simulink model "controller"  (R2021a)
settings: Solver=FixedStepDiscrete  StartTime=0.0  StopTime=10.0  FixedStep=1  RelTol=1e-3  EnableMultiTasking=on
settings Model: DataDictionary=worldDD.sldd  SILPILModeSetting=veronly  ExtModeTrigDuration=2  Creator=Koorosh  LastModifiedBy=Koorosh
settings OptimizationCC: EnhancedBackFolding=on  PassReuseOutputArgsAs=Individual arguments  ZeroExternalMemoryAtStartup=off  ZeroInternalMemoryAtStartup=off  MaxStackSize=64  OptimizeBlockOrder=speed  DifferentSizesBufferReuse=on  OptimizationCustomize=off  EfficientTunableParamExpr=on
settings DebuggingCC: ParameterTunabilityLossMsg=error
settings HardwareCC: ProdBitPerInt=16  ProdBitPerPointer=16  ProdBitPerSizeT=16  ProdBitPerPtrDiffT=16  ProdLargestAtomicFloat=None  ProdWordSize=8  ProdHWDeviceType=Atmel->AVR
settings SFSimCC: MATLABDynamicMemAlloc=off
settings RTWCC: SystemTargetFile=ert.tlc  HardwareBoard=Arduino Uno  GenCodeOnly=on  TemplateMakefile=ert_default_tmf  GenerateReport=on  Toolchain=Arduino AVR  BuildConfiguration=Faster Runs  LaunchReport=on  GenerateWebview=on
settings CodeAppCC: ForceParamTrailComments=on  IgnoreCustomStorageClasses=off  OperatorAnnotations=on  SimulinkDataObjDesc=on  SFDataObjDesc=on  InsertBlockDesc=on
settings ERTTargetCC: SupportContinuousTime=on  SupportVariableSizeSignals=on  ExtModeStaticAllocSize=250

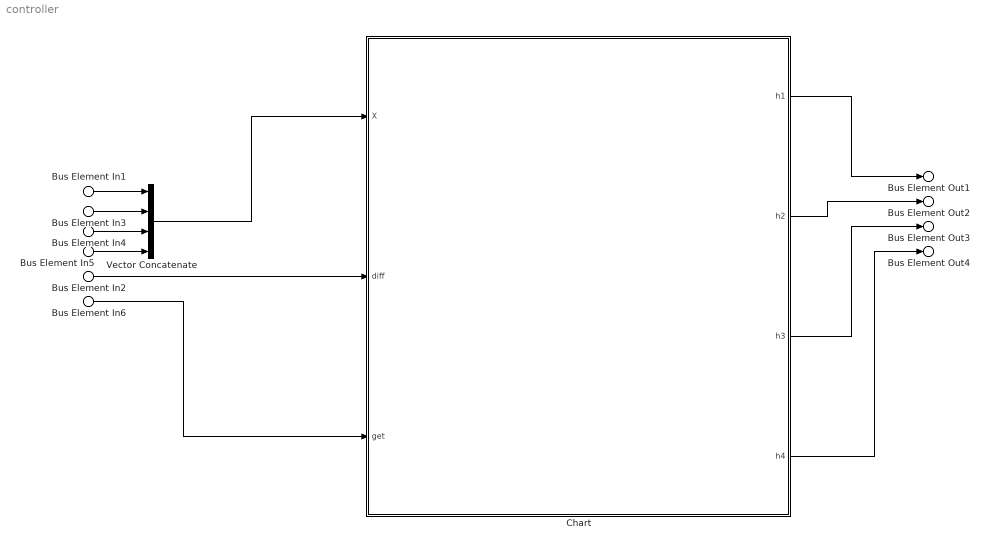
== system controller ==
  Bus Element In1 : Inport  PortName=X  Element=x1
  Bus Element In3 : Inport  PortName=X  Element=x2
  Bus Element In4 : Inport  PortName=X  Element=x3
  Bus Element In5 : Inport  PortName=X  Element=x4
  Bus Element In6 : Inport  Port=2  PortName=C  Element=get
  Bus Element In2 : Inport  Port=2  PortName=C  Element=diff
  Chart : Stateflow chart  TreatAsAtomicUnit=on
  Vector Concatenate : Concatenate  NumInputs=4
  Bus Element Out1 : Outport  PortName=H  Element=h1
  Bus Element Out2 : Outport  PortName=H  Element=h2
  Bus Element Out3 : Outport  PortName=H  Element=h3
  Bus Element Out4 : Outport  PortName=H  Element=h4
  wires:
  Chart/1(h1) -> Bus Element Out1/1
  Chart/2(h2) -> Bus Element Out2/1
  Chart/3(h3) -> Bus Element Out3/1
  Chart/4(h4) -> Bus Element Out4/1
  Bus Element In2/1 -> Chart/2(diff)
  Bus Element In6/1 -> Chart/3(get)
  Bus Element In1/1 -> Vector Concatenate/1
  Bus Element In3/1 -> Vector Concatenate/2
  Bus Element In4/1 -> Vector Concatenate/3
  Bus Element In5/1 -> Vector Concatenate/4
  Vector Concatenate/1 -> Chart/1(X)

== stateflow chart controller/Chart ==
  settings: stateMachineType=MOORE_MACHINE
  state h1h2
    U(1,2);
  state h1h3
    U(1,3);
  state init_state
  state h1h4
    U(1,4);
  state h3h4
    U(3,4);
  state h2h3
    U(2,3);
  state h2h4
    U(2,4);
  h1h2 -> h3h4 [order 2] : [(T(1,3)&T(2,4))|(T(1,4)&T(2,3))]
  h1h3 -> h1h2 [order 1] : [T(3,2)|(T(1,2)&T(3,1))]
  h1h3 -> h1h4 [order 2] : [T(3,4)|(T(1,4)&T(3,1))]
  h1h2 -> h1h3 [order 1] : [T(2,3)|(T(2,1)&T(1,3))]
  h1h4 -> h1h2 [order 4] : [T(4,2)|(T(1,2)&T(4,1))]
  h3h4 -> h1h2 [order 2] : [(T(3,1)&T(4,2))|(T(4,1)&T(3,2))]
  h1h4 -> h1h3 [order 1] : [T(4,3)|(T(4,1)&T(1,3))]
  h3h4 -> h1h3 [order 4] : [T(4,1)|(T(4,3)&T(3,1))]
  h1h2 -> h1h4 [order 5] : [T(2,4)|(T(2,1)&T(1,4))]
  h1h3 -> h3h4 [order 5] : [T(1,4)|(T(3,4)&T(1,3))]
  h2h3 -> h1h2 [order 4] : [T(3,1)|(T(2,1)&T(3,2))]
  h1h2 -> h2h3 [order 4] : [T(1,3)|(T(1,2)&T(2,3))]
  init_state -> h1h2 [order 1] : [h1==1 & h2==1]
  h2h4 -> h1h2 [order 3] : [T(4,1)|(T(2,1)&T(4,2))]
  h1h2 -> h2h4 [order 3] : [T(1,4)|(T(1,2)&T(2,4))]
  h2h3 -> h1h3 [order 3] : [T(2,1)|(T(3,1)&T(2,3))]
  h1h3 -> h2h3 [order 3] : [T(1,2)|(T(1,3)&T(3,2))]
  init_state -> h1h3 [order 2] : [h1==1 & h3==1]
  h2h4 -> h1h3 [order 4] : [(T(2,1)&T(4,3))|(T(4,1)&T(2,3))]
  h1h3 -> h2h4 [order 4] : [(T(1,2)&T(3,4))|(T(1,4)&T(3,2))]
  (default) -> init_state
  h1h4 -> h3h4 [order 3] : [T(1,3)|(T(1,4)&T(4,3))]
  init_state -> h3h4 [order 4] : [h3==1 & h4==1]
  init_state -> h1h4 [order 3] : [h1==1 & h4==1]
  h3h4 -> h1h4 [order 3] : [T(3,1)|(T(4,1)&T(3,4))]
  h2h3 -> h1h4 [order 1] : [(T(2,1)&T(3,4))|(T(2,4)&T(3,1))]
  h1h4 -> h2h3 [order 2] : [(T(1,2)&T(4,3))|(T(4,2)&T(1,3))]
  h2h4 -> h1h4 [order 5] : [T(2,1)|(T(4,1)&T(2,4))]
  h1h4 -> h2h4 [order 5] : [T(1,2)|(T(1,4)&T(4,2))]
  h2h3 -> h3h4 [order 5] : [T(2,4)|(T(2,3)&T(3,4))]
  h3h4 -> h2h3 [order 5] : [T(4,2)|(T(3,2)&T(4,3))]
  h2h4 -> h3h4 [order 2] : [T(2,3)|(T(2,4)&T(4,3))]
  h3h4 -> h2h4 [order 1] : [T(3,2)|(T(4,2)&T(3,4))]
  init_state -> h2h3 [order 5] : [h2==1 & h3==1]
  init_state -> h2h4 [order 6] : [h2==1 & h4==1]
  h2h3 -> h2h4 [order 2] : [T(3,4)|(T(2,4)&T(3,2))]
  h2h4 -> h2h3 [order 1] : [T(4,3)|(T(4,2)&T(2,3))]
  data: i function_input; condition function_output; j function_input; i1 function_input; i2 function_input; X input; h1 output =int8(0); h2 output =int8(1); h3 output =int8(1); h4 output =int8(0); diff input; get input
  function condition = T(i,j):
    | function condition = T(i,j)
    |     condition = (X(j)<=get(j))&((X(i)-X(j))>=diff(j));
    | end
  function U(i1,i2):
    | function U(i1,i2)
    |     [h1,h2,h3,h4]=deal(int8(0),int8(0),int8(0),int8(0));
    |     if((i1==1)||(i2==1))
    |         h1=int8(1);
    |     end    
    |     if((i1==2)||(i2==2))
    |         h2=int8(1);
    |     end
    |     if((i1==3)||(i2==3))
    |         h3=int8(1);
    |     end
    |     if((i1==4)||(i2==4))
    |         h4=int8(1);
    |     end
    | end
